simulink model "Final"  (R2017b)
settings: Solver=VariableStepAuto  StartTime=0.0  StopTime=50  RelTol=1e-3
values from neighbouring files (symbols this model uses):
  kd = eval(S.kd)    [Lab4.m]    (also in Lab4Final.m; Lab4intento2.m; Lab4intento3.m)
  kd2 = eval(S.kd2)    [Lab4.m]    (also in Lab4Final.m; Lab4intento3.m)
  ki = eval(S.ki)    [Lab4.m]    (also in Lab4Final.m; Lab4intento2.m; Lab4intento3.m)
  kp = eval(S.kp)    [Lab4.m]    (also in Lab4Final.m; Lab4intento2.m; Lab4intento3.m)
libraries: simulink x1
settings Model: Creator=Cx001la  LastModifiedBy=Cx001la

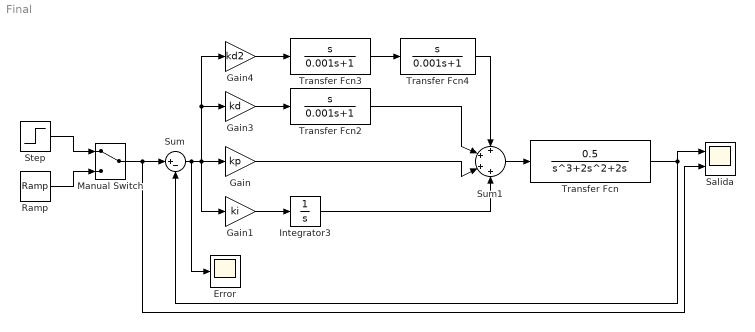
== system Final ==
  Error : Scope
  Gain : Gain  Gain=kp
  Gain1 : Gain  Gain=ki
  Gain3 : Gain  Gain=kd
  Gain4 : Gain  Gain=kd2
  Integrator3 : Integrator
  Manual Switch : ManualSwitch
  Ramp : simulink/Sources/Ramp  slope=1  start=0  X0=0
  Salida : Scope  NumInputPorts=2
  Step : Step  Time=0  SampleTime=0
  Sum : Sum  Inputs=|+-
  Sum1 : Sum  Inputs=++++
  Transfer Fcn : TransferFcn  Numerator=[0.5]  Denominator=[1 2 2 0]
  Transfer Fcn2 : TransferFcn  Numerator=[1 0]  Denominator=[0.001 1]
  Transfer Fcn3 : TransferFcn  Numerator=[1 0]  Denominator=[0.001 1]
  Transfer Fcn4 : TransferFcn  Numerator=[1 0]  Denominator=[0.001 1]
  wires:
  Sum/1 -> Error/1, Gain1/1, Gain4/1, Gain3/1, Gain/1
  Gain1/1 -> Integrator3/1
  Gain4/1 -> Transfer Fcn3/1
  Gain3/1 -> Transfer Fcn2/1
  Gain/1 -> Sum1/3
  Transfer Fcn2/1 -> Sum1/2
  Transfer Fcn4/1 -> Sum1/1
  Integrator3/1 -> Sum1/4
  Sum1/1 -> Transfer Fcn/1
  Transfer Fcn/1 -> Sum/2, Salida/1
  Transfer Fcn3/1 -> Transfer Fcn4/1
  Step/1 -> Manual Switch/1
  Manual Switch/1 -> Salida/2, Sum/1
  Ramp/1 -> Manual Switch/2
